simulink model "sysgenDDC"  (Simulink 7.7)
settings: Solver=VariableStepDiscrete  SolverMode=SingleTasking  StartTime=0.0  StopTime=0.003  RelTol=1e-3
PreLoadFcn:
  | sysgenDDC_PreLoadFcn
values from neighbouring files (symbols this model uses):
  Gz = [  340 ... (first row only)    [sysgenDDC_PreLoadFcn.m]
  Hz = [479 ... (first row only)    [sysgenDDC_PreLoadFcn.m]
  Ts = 1/40e006    (= 2.5e-08)    [sysgenDDC_PreLoadFcn.m]
undefined symbols (not defined in the file or in its folder): get, One, sided, xlGetSimulinkPeriod, xlipgetpartsetting
libraries: xbsIndex_r4 x132, dspsnks4 x2, xbsCopyrightNotice_r4 x1
(part 2 of 2)

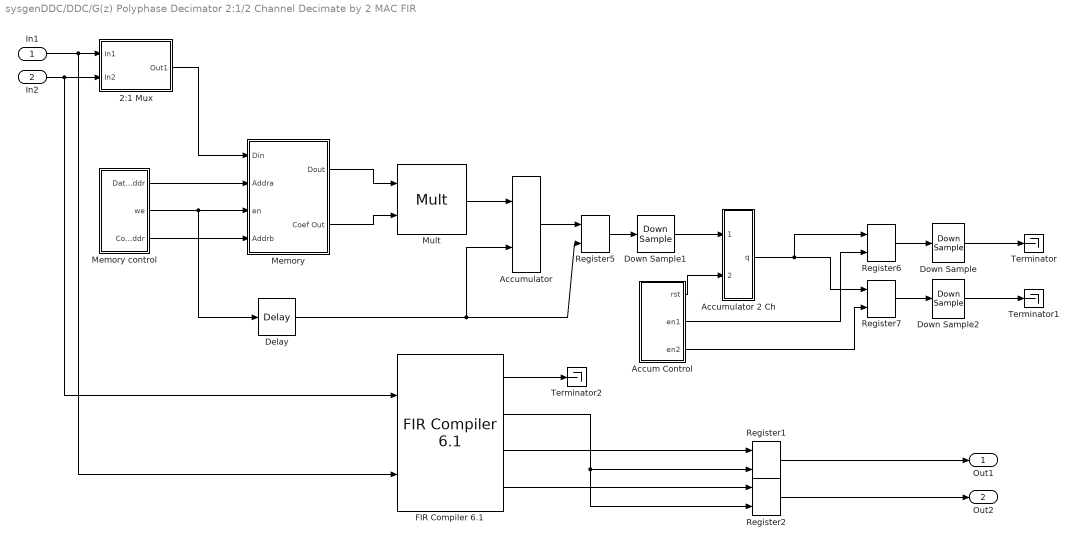
== system sysgenDDC/DDC/G(z) Polyphase Decimator 2:1/2 Channel Decimate by 2 MAC FIR  ==
  In1 : Inport
  In2 : Inport  Port=2
  2:1 Mux : Subsystem
  Accum Control : Subsystem
  Accumulator : xbsIndex_r4/Accumulator  operation=Add  n_bits=ceil(log2(coef_sum*(2^(bit_width-1))))  overflow=Wrap  scale=1  rst=on  hasbypass=on  en=off  dbl_ovrd=off  use_behavioral_HDL=on  implementation=Fabric  block_type=accum
      settings: infoedit="Adder or subtractor-based accumulator.   Output type and binary point position match the input.<P><P>Hardware notes: When \"Reinitialize with input 'b' on reset\" is selected, the accumulator is forced to run at the system rate even if the input 'b' is running at a slower rate."  xl_area=[18 36 0 36 0 0 0]  block_version=VER_STRING_GOES_HERE
  Accumulator 2 Ch : Subsystem
  Delay : xbsIndex_r4/Delay  rst=off  infoeditControl=Selection of Reset will increase slice count due to use of real FFs and instead of SRLs  en=off  latency=3  dbl_ovrd=off  reg_retiming=off  block_type=delay
      settings: infoedit=Hardware notes: A delay line is a chain, each link of which is an SRL16 followed by a flip-flop. If register retiming is enabled, the delay line is a chain of flip-flops.  xl_area=[1 1 0 1 0 0 0]  block_version=VER_STRING_GOES_HERE
  Down Sample : xbsIndex_r4/Down Sample  sample_ratio=4  sample_phase="Last Value of Frame  (most efficient)"  en=off  latency=1  dbl_ovrd=off  block_type=dsamp
      settings: xl_area=[19 37 0 0 0 0 0]  block_version=VER_STRING_GOES_HERE
  Down Sample1 : xbsIndex_r4/Down Sample  sample_ratio=length(coef)/4  sample_phase="Last Value of Frame  (most efficient)"  en=off  latency=1  dbl_ovrd=off  block_type=dsamp
      settings: xl_area=[18 36 0 0 0 0 0]  block_version=VER_STRING_GOES_HERE
  Down Sample2 : xbsIndex_r4/Down Sample  sample_ratio=4  sample_phase="Last Value of Frame  (most efficient)"  en=off  latency=1  dbl_ovrd=off  block_type=dsamp
      settings: xl_area=[19 37 0 0 0 0 0]  block_version=VER_STRING_GOES_HERE
  "FIR Compiler 6.1 " : xbsIndex_r4/FIR Compiler 6.1   coefficientvector=Gz  coefficient_sets=1  filter_type=Decimation  rate_change_type=Integer  interpolation_rate=1  decimation_rate=2  number_channels=1  ratespecification=Maximum_Possible  sampleperiod=96  hardwareoversamplingrate=1  coefficient_reload=off  coefficient_sign=Signed  quantization=Integer_Coefficients  coefficient_width=18  bestprecision=off  coefficient_fractional_bits=0  coefficient_structure=Inferred  number_paths=2  output_rounding_mode=Full_Precision  output_width=36  optimization_goal=Area  data_has_tlast=Not_Required  m_data_has_tready=off  s_data_has_tuser=Not_Required  m_data_has_tuser=Not_Required  s_config_sync_mode=On_Vector  s_config_method=Single  num_reload_slots=1  has_aclken=off  has_aresetn=off  multi_column_support=Disabled  columnconfig='7'  inter_column_pipe_length=4  data_buffer_type=Automatic  coefficient_buffer_type=Automatic  input_buffer_type=Automatic  output_buffer_type=Automatic  preference_for_other_storage=Automatic  trim_axipin_name=on  passband_min=0.0  passband_max=0.5  stopband_min=0.5  stopband_max=1.0  filter_selection=1  gui_behaviour=Sysgen_GUI  data_sign=Signed  data_width=16  data_fractional_bits=0  wrapper_available=true  ip_wrap_arbitrary_binary_point=true  ip_name=FIR Compiler  ip_version=6.1  dsptool_ready=true  ipcore_usecache=true  ipcore_useipmodelcache=true  ipcore_xco_need_fpga_part=true  port_translation_map={ 'aclken' => 'en', 'aresetn' => 'rst' }  run_core_at_system_period=true  ipcore_fpga_part=xlipgetpartsetting(gcb, {'virtex6', 'xc6vlx75t', '-3', 'ff784'})  structural_sim=false  block_type=fir_compiler_v6_1
      settings: infoedit=Maximum Possible : Maximizes oversampling rate. Abtracted input handshake (no s_data_tvalid) and automatic rate propagation.<br><br>Hardware Oversampling Rate : Specifies oversampling rate relative to the input sample period. Abtracted input handshake (no s_data_tvalid) and automatic rate propagation.<br><br>Sample Period : Specifies absolute oversampling rate. No input handshake abstraction (exposes s_data_tvalid) and no rate propagation.
  Memory : Subsystem
  Memory control : Subsystem
  Mult : xbsIndex_r4/Mult  precision=Full  arith_type="Signed  (2's comp)"  n_bits=8  bin_pt=2  quantization=Truncate  overflow=Wrap  en=off  latency=1  dbl_ovrd=off  use_behavioral_HDL=off  opt=Speed  use_embedded=on  optimum_pipeline=off  pipeline=on  use_rpm=off  placement_style=Rectangular shape  block_type=mult
      settings: infoedit=Hardware notes: To use the internal pipeline stage of the dedicated multiplier you must select 'Pipeline to Greatest Extent Possible'.  xl_area=[0 0 0 0 0 1 0]  block_version=VER_STRING_GOES_HERE
  Register{1..2,5..7} (5 alike) : xbsIndex_r4/Register  init=0  rst=off  en=on  dbl_ovrd=off  block_type=register
      Register1 settings: xl_area=[19 37 0 0 0 0 0]  block_version=VER_STRING_GOES_HERE
      Register2 settings: xl_area=[19 37 0 0 0 0 0]  block_version=VER_STRING_GOES_HERE
      Register5 settings: xl_area=[18 36 0 0 0 0 0]  block_version=VER_STRING_GOES_HERE
      Register6 settings: xl_area=[19 37 0 0 0 0 0]  block_version=VER_STRING_GOES_HERE
      Register7 settings: xl_area=[19 37 0 0 0 0 0]  block_version=VER_STRING_GOES_HERE
  Terminator : Terminator
  Terminator1 : Terminator
  Terminator2 : Terminator
  Out1 : Outport
  Out2 : Outport  Port=2
  wires:
  In2/1 -> 2:1 Mux/2(In2), "FIR Compiler 6.1 "/1
  Accum Control/3(en2) -> Register7/2
  Accum Control/2(en1) -> Register6/2
  Accum Control/1(rst) -> Accumulator 2 Ch/2(rst)
  Register7/1 -> Down Sample2/1
  Accumulator 2 Ch/1(q) -> Register6/1, Register7/1
  Register6/1 -> Down Sample/1
  Register5/1 -> Down Sample1/1
  Accumulator/1 -> Register5/1
  Memory control/3(Coef Addr) -> Memory/4(Addrb)
  Memory control/2(we) -> Delay/1, Memory/3(en)
  Memory control/1(Data Addr) -> Memory/2(Addra)
  Memory/1(Dout) -> Mult/1
  Mult/1 -> Accumulator/1
  Delay/1 -> Accumulator/2, Register5/2
  Down Sample1/1 -> Accumulator 2 Ch/1(In)
  Memory/2(Coef Out) -> Mult/2
  2:1 Mux/1(Out1) -> Memory/1(Din)
  In1/1 -> 2:1 Mux/1(In1), "FIR Compiler 6.1 "/2
  Register1/1 -> Out1/1
  Register2/1 -> Out2/1
  "FIR Compiler 6.1 "/4 -> Register2/1
  "FIR Compiler 6.1 "/3 -> Register1/1
  "FIR Compiler 6.1 "/2 -> Register1/2, Register2/2
  Down Sample/1 -> Terminator/1
  Down Sample2/1 -> Terminator1/1
  "FIR Compiler 6.1 "/1 -> Terminator2/1

== system sysgenDDC/DDC/G(z) Polyphase Decimator 2:1/Symmetric Round2 ==
  data : Inport
  Convert : xbsIndex_r4/Convert  gui_display_data_type=Fixed-point  arith_type="Signed  (2's comp)"  n_bits=18  bin_pt=0  float_type=Single  exp_bits=8  fraction_bits=24  quantization="Round  (unbiased: +/- Inf)"  overflow=Flag as error  en=off  latency=0  dbl_ovrd=off  pipeline=off  block_type=convert
      settings: xl_area=[13 0 0 25 0 0 0]  block_version=VER_STRING_GOES_HERE
  Reinterpret : xbsIndex_r4/Reinterpret  force_arith_type=off  arith_type="Signed  (2's comp)"  force_bin_pt=on  bin_pt=38-18  block_type=cast
      settings: infoedit="Changes signal type without altering the binary representation.   You can changed the signal between signed and unsigned, and relocate the binary point.<br><br>Hardware notes: In hardware this block costs nothing.<br><br>Example:  Suppose the input is 6 bits wide, signed, with 2 fractional bits, and the output is forced to unsigned with 0 fractional bits.  Then an input of -2.0 (1110.00 in binary 2's complement) becomes an output of 56 (111000 in binary)."  block_version=VER_STRING_GOES_HERE
  " out" : Outport
  wires:
  Reinterpret/1 -> Convert/1
  data/1 -> Reinterpret/1
  Convert/1 -> " out"/1

== system sysgenDDC/DDC/G(z) Polyphase Decimator 2:1/Symmetric Round3 ==
  data : Inport
  Convert : xbsIndex_r4/Convert  gui_display_data_type=Fixed-point  arith_type="Signed  (2's comp)"  n_bits=18  bin_pt=0  float_type=Single  exp_bits=8  fraction_bits=24  quantization="Round  (unbiased: +/- Inf)"  overflow=Flag as error  en=off  latency=0  dbl_ovrd=off  pipeline=off  block_type=convert
      settings: xl_area=[13 0 0 25 0 0 0]  block_version=VER_STRING_GOES_HERE
  Reinterpret : xbsIndex_r4/Reinterpret  force_arith_type=off  arith_type="Signed  (2's comp)"  force_bin_pt=on  bin_pt=38-18  block_type=cast
      settings: infoedit="Changes signal type without altering the binary representation.   You can changed the signal between signed and unsigned, and relocate the binary point.<br><br>Hardware notes: In hardware this block costs nothing.<br><br>Example:  Suppose the input is 6 bits wide, signed, with 2 fractional bits, and the output is forced to unsigned with 0 fractional bits.  Then an input of -2.0 (1110.00 in binary 2's complement) becomes an output of 56 (111000 in binary)."  block_version=VER_STRING_GOES_HERE
  " out" : Outport
  wires:
  Reinterpret/1 -> Convert/1
  Convert/1 -> " out"/1
  data/1 -> Reinterpret/1

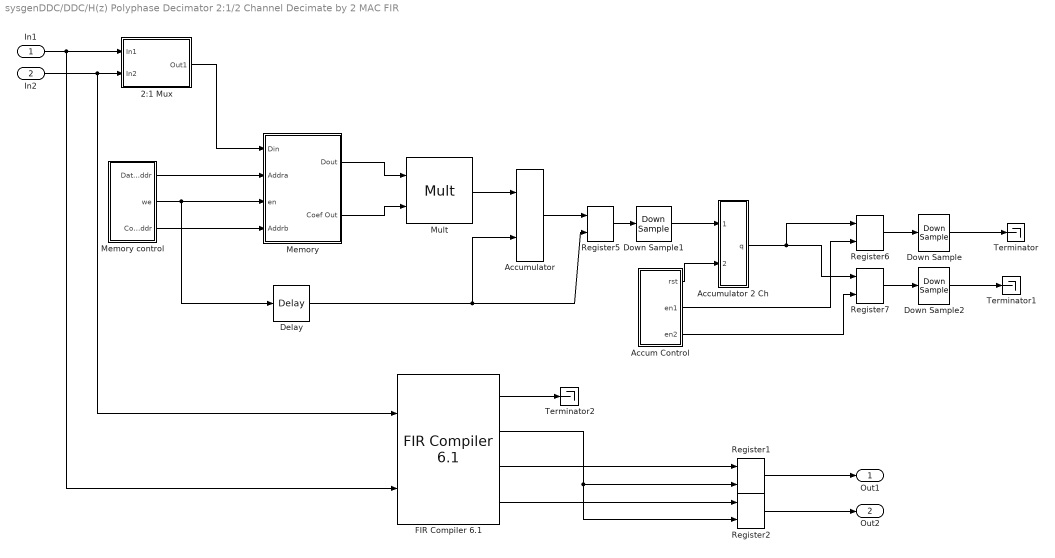
== system sysgenDDC/DDC/H(z) Polyphase Decimator 2:1/2 Channel Decimate by 2 MAC FIR  ==
  In1 : Inport
  In2 : Inport  Port=2
  2:1 Mux : Subsystem
  Accum Control : Subsystem
  Accumulator : xbsIndex_r4/Accumulator  operation=Add  n_bits=ceil(log2(coef_sum*(2^(bit_width-1))))  overflow=Wrap  scale=1  rst=on  hasbypass=on  en=off  dbl_ovrd=off  use_behavioral_HDL=on  implementation=Fabric  block_type=accum
      settings: infoedit="Adder or subtractor-based accumulator.   Output type and binary point position match the input.<P><P>Hardware notes: When \"Reinitialize with input 'b' on reset\" is selected, the accumulator is forced to run at the system rate even if the input 'b' is running at a slower rate."  xl_area=[18 36 0 36 0 0 0]  block_version=VER_STRING_GOES_HERE
  Accumulator 2 Ch : Subsystem
  Delay : xbsIndex_r4/Delay  rst=off  infoeditControl=Selection of Reset will increase slice count due to use of real FFs and instead of SRLs  en=off  latency=4  dbl_ovrd=off  reg_retiming=off  block_type=delay
      settings: infoedit=Hardware notes: A delay line is a chain, each link of which is an SRL16 followed by a flip-flop. If register retiming is enabled, the delay line is a chain of flip-flops.  xl_area=[1 1 0 1 0 0 0]  block_version=VER_STRING_GOES_HERE
  Down Sample : xbsIndex_r4/Down Sample  sample_ratio=4  sample_phase="Last Value of Frame  (most efficient)"  en=off  latency=1  dbl_ovrd=off  block_type=dsamp
      settings: xl_area=[19 37 0 0 0 0 0]  block_version=VER_STRING_GOES_HERE
  Down Sample1 : xbsIndex_r4/Down Sample  sample_ratio=length(coef)/4  sample_phase="Last Value of Frame  (most efficient)"  en=off  latency=1  dbl_ovrd=off  block_type=dsamp
      settings: xl_area=[18 36 0 0 0 0 0]  block_version=VER_STRING_GOES_HERE
  Down Sample2 : xbsIndex_r4/Down Sample  sample_ratio=4  sample_phase="Last Value of Frame  (most efficient)"  en=off  latency=1  dbl_ovrd=off  block_type=dsamp
      settings: xl_area=[19 37 0 0 0 0 0]  block_version=VER_STRING_GOES_HERE
  "FIR Compiler 6.1 " : xbsIndex_r4/FIR Compiler 6.1   coefficientvector=Hz  coefficient_sets=1  filter_type=Decimation  rate_change_type=Integer  interpolation_rate=1  decimation_rate=2  number_channels=1  ratespecification=Maximum_Possible  sampleperiod=96  hardwareoversamplingrate=1  coefficient_reload=off  coefficient_sign=Signed  quantization=Integer_Coefficients  coefficient_width=18  bestprecision=off  coefficient_fractional_bits=0  coefficient_structure=Inferred  number_paths=2  output_rounding_mode=Full_Precision  output_width=36  optimization_goal=Area  data_has_tlast=Not_Required  m_data_has_tready=off  s_data_has_tuser=Not_Required  m_data_has_tuser=Not_Required  s_config_sync_mode=On_Vector  s_config_method=Single  num_reload_slots=1  has_aclken=off  has_aresetn=off  multi_column_support=Disabled  columnconfig='26'  inter_column_pipe_length=4  data_buffer_type=Automatic  coefficient_buffer_type=Automatic  input_buffer_type=Automatic  output_buffer_type=Automatic  preference_for_other_storage=Automatic  trim_axipin_name=on  passband_min=0.0  passband_max=0.5  stopband_min=0.5  stopband_max=1.0  filter_selection=1  gui_behaviour=Sysgen_GUI  data_sign=Signed  data_width=16  data_fractional_bits=0  wrapper_available=true  ip_wrap_arbitrary_binary_point=true  ip_name=FIR Compiler  ip_version=6.1  dsptool_ready=true  ipcore_usecache=true  ipcore_useipmodelcache=true  ipcore_xco_need_fpga_part=true  port_translation_map={ 'aclken' => 'en', 'aresetn' => 'rst' }  run_core_at_system_period=true  ipcore_fpga_part=xlipgetpartsetting(gcb, {'virtex6', 'xc6vlx75t', '-3', 'ff784'})  structural_sim=false  block_type=fir_compiler_v6_1
      settings: infoedit=Maximum Possible : Maximizes oversampling rate. Abtracted input handshake (no s_data_tvalid) and automatic rate propagation.<br><br>Hardware Oversampling Rate : Specifies oversampling rate relative to the input sample period. Abtracted input handshake (no s_data_tvalid) and automatic rate propagation.<br><br>Sample Period : Specifies absolute oversampling rate. No input handshake abstraction (exposes s_data_tvalid) and no rate propagation.
  Memory : Subsystem
  Memory control : Subsystem
  Mult : xbsIndex_r4/Mult  precision=Full  arith_type="Signed  (2's comp)"  n_bits=8  bin_pt=2  quantization=Truncate  overflow=Wrap  en=off  latency=2  dbl_ovrd=off  use_behavioral_HDL=off  opt=Speed  use_embedded=on  optimum_pipeline=off  pipeline=on  use_rpm=off  placement_style=Rectangular shape  block_type=mult
      settings: infoedit=Hardware notes: To use the internal pipeline stage of the dedicated multiplier you must select 'Pipeline to Greatest Extent Possible'.  xl_area=[18 36 0 0 0 1 0]  block_version=VER_STRING_GOES_HERE
  Register{1..2,5..7} (5 alike) : xbsIndex_r4/Register  init=0  rst=off  en=on  dbl_ovrd=off  block_type=register
      Register1 settings: xl_area=[19 37 0 0 0 0 0]  block_version=VER_STRING_GOES_HERE
      Register2 settings: xl_area=[19 37 0 0 0 0 0]  block_version=VER_STRING_GOES_HERE
      Register5 settings: xl_area=[18 36 0 0 0 0 0]  block_version=VER_STRING_GOES_HERE
      Register6 settings: xl_area=[19 37 0 0 0 0 0]  block_version=VER_STRING_GOES_HERE
      Register7 settings: xl_area=[19 37 0 0 0 0 0]  block_version=VER_STRING_GOES_HERE
  Terminator : Terminator
  Terminator1 : Terminator
  Terminator2 : Terminator
  Out1 : Outport
  Out2 : Outport  Port=2
  wires:
  In1/1 -> 2:1 Mux/1(In1), "FIR Compiler 6.1 "/2
  2:1 Mux/1(Out1) -> Memory/1(Din)
  Memory/2(Coef Out) -> Mult/2
  Down Sample1/1 -> Accumulator 2 Ch/1(In)
  Delay/1 -> Register5/2, Accumulator/2
  Mult/1 -> Accumulator/1
  Memory/1(Dout) -> Mult/1
  Memory control/1(Data Addr) -> Memory/2(Addra)
  Memory control/2(we) -> Memory/3(en), Delay/1
  Memory control/3(Coef Addr) -> Memory/4(Addrb)
  Accumulator/1 -> Register5/1
  Register5/1 -> Down Sample1/1
  Register6/1 -> Down Sample/1
  Accumulator 2 Ch/1(q) -> Register7/1, Register6/1
  Register7/1 -> Down Sample2/1
  Accum Control/1(rst) -> Accumulator 2 Ch/2(rst)
  Accum Control/2(en1) -> Register6/2
  Accum Control/3(en2) -> Register7/2
  In2/1 -> 2:1 Mux/2(In2), "FIR Compiler 6.1 "/1
  "FIR Compiler 6.1 "/4 -> Register2/1
  "FIR Compiler 6.1 "/3 -> Register1/1
  "FIR Compiler 6.1 "/2 -> Register1/2, Register2/2
  Register1/1 -> Out1/1
  Register2/1 -> Out2/1
  Down Sample/1 -> Terminator/1
  Down Sample2/1 -> Terminator1/1
  "FIR Compiler 6.1 "/1 -> Terminator2/1

== system sysgenDDC/DDC/H(z) Polyphase Decimator 2:1/Coarse Gain ==
  data : Inport
  Reinterpret : xbsIndex_r4/Reinterpret  force_arith_type=on  arith_type="Signed  (2's comp)"  force_bin_pt=on  bin_pt=24  block_type=cast
      settings: infoedit="Changes type of samples without altering their binary representation.<P><P>Hardware notes: In hardware this block costs nothing.<P><P>Example:  Suppose the input is 6 bits wide, signed, with 2 fractional bits, and the output is forced to unsigned with 0 fractional bits.  Then an input of -2.0 (1110.00 in binary 2's complement) becomes an output of 56 (111000 in binary)."  block_version=VER_STRING_GOES_HERE
  Slice : xbsIndex_r4/Slice  nbits=26  boolean_output=off  mode=Upper Bit Location + Width  bit1=0  base1=MSB of Input  bit0=0  base0=LSB of Input  dbl_ovrd=off  block_type=slice
      settings: infoedit="Extracts a given range of bits from each input sample and presents it at the output.  The output type is ordinarily unsigned with binary point at zero, but can be Boolean when the slice is one bit wide.<P><P>Hardware notes: In hardware this block costs nothing."  block_version=VER_STRING_GOES_HERE
  " out" : Outport
  wires:
  Reinterpret/1 -> " out"/1
  Slice/1 -> Reinterpret/1
  data/1 -> Slice/1

== system sysgenDDC/DDC/H(z) Polyphase Decimator 2:1/Coarse Gain1 ==
  data : Inport
  Reinterpret : xbsIndex_r4/Reinterpret  force_arith_type=on  arith_type="Signed  (2's comp)"  force_bin_pt=on  bin_pt=24  block_type=cast
      settings: infoedit="Changes type of samples without altering their binary representation.<P><P>Hardware notes: In hardware this block costs nothing.<P><P>Example:  Suppose the input is 6 bits wide, signed, with 2 fractional bits, and the output is forced to unsigned with 0 fractional bits.  Then an input of -2.0 (1110.00 in binary 2's complement) becomes an output of 56 (111000 in binary)."  block_version=VER_STRING_GOES_HERE
  Slice : xbsIndex_r4/Slice  nbits=26  boolean_output=off  mode=Upper Bit Location + Width  bit1=0  base1=MSB of Input  bit0=0  base0=LSB of Input  dbl_ovrd=off  block_type=slice
      settings: infoedit="Extracts a given range of bits from each input sample and presents it at the output.  The output type is ordinarily unsigned with binary point at zero, but can be Boolean when the slice is one bit wide.<P><P>Hardware notes: In hardware this block costs nothing."  block_version=VER_STRING_GOES_HERE
  " out" : Outport
  wires:
  data/1 -> Slice/1
  Slice/1 -> Reinterpret/1
  Reinterpret/1 -> " out"/1

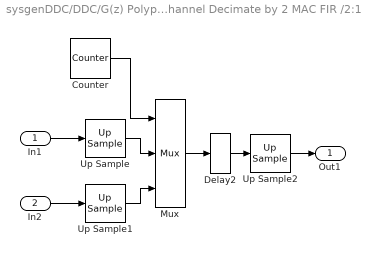
== system sysgenDDC/DDC/G(z) Polyphase Decimator 2:1/2 Channel Decimate by 2 MAC FIR /2:1 Mux ==
  In1 : Inport
  In2 : Inport  Port=2
  Counter : xbsIndex_r4/Counter  cnt_type=Free Running  cnt_to=Inf  operation=Up  start_count=0  cnt_by_val=1  arith_type=Unsigned  n_bits=1  bin_pt=0  load_pin=off  rst=off  en=off  explicit_period=off  period=Ts/2  dbl_ovrd=off  use_behavioral_HDL=off  implementation=Fabric  use_rpm=off  block_type=counter
      settings: xl_area=[2 1 0 1 0 0 0]  block_version=VER_STRING_GOES_HERE
  Delay2 : xbsIndex_r4/Delay  rst=off  infoeditControl=Selection of Reset will increase slice count due to use of real FFs and instead of SRLs  en=off  latency=1  dbl_ovrd=off  reg_retiming=off  block_type=delay
      settings: infoedit=Hardware notes: A delay line is a chain, each link of which is an SRL16 followed by a flip-flop. If register retiming is enabled, the delay line is a chain of flip-flops.  xl_area=[9 18 0 0 0 0 0]  block_version=VER_STRING_GOES_HERE
  Mux : xbsIndex_r4/Mux  inputs=2  en=off  latency=0  precision=Full  arith_type="Signed  (2's comp)"  n_bits=8  bin_pt=2  quantization=Truncate  overflow=Wrap  dbl_ovrd=off  block_type=mux
      settings: xl_area=[9 0 0 18 0 0 0]  block_version=VER_STRING_GOES_HERE
  Up Sample : xbsIndex_r4/Up Sample  sample_ratio=2  copy_samples=on  en=off  latency=0  dbl_ovrd=off  block_type=usamp
      settings: infoedit="Up samples input data.  Inserted values  can be zeros or copies of the most recent input sample.<P><P>Hardware notes: No hardware is needed if inserted values are copies of the input sample; otherwise, a mux and single bit flip-flop are used."  xl_area=[0 0 0 0 0 0 0]  block_version=VER_STRING_GOES_HERE
  Up Sample1 : xbsIndex_r4/Up Sample  sample_ratio=2  copy_samples=on  en=off  latency=0  dbl_ovrd=off  block_type=usamp
      settings: infoedit="Up samples input data.  Inserted values  can be zeros or copies of the most recent input sample.<P><P>Hardware notes: No hardware is needed if inserted values are copies of the input sample; otherwise, a mux and single bit flip-flop are used."  xl_area=[0 0 0 0 0 0 0]  block_version=VER_STRING_GOES_HERE
  Up Sample2 : xbsIndex_r4/Up Sample  sample_ratio=length(coef)/4  copy_samples=on  en=off  latency=0  dbl_ovrd=off  block_type=usamp
      settings: infoedit="Up samples input data.  Inserted values  can be zeros or copies of the most recent input sample.<P><P>Hardware notes: No hardware is needed if inserted values are copies of the input sample; otherwise, a mux and single bit flip-flop are used."  xl_area=[0 0 0 0 0 0 0]  block_version=VER_STRING_GOES_HERE
  Out1 : Outport
  wires:
  Up Sample2/1 -> Out1/1
  In2/1 -> Up Sample1/1
  In1/1 -> Up Sample/1
  Delay2/1 -> Up Sample2/1
  Mux/1 -> Delay2/1
  Counter/1 -> Mux/1
  Up Sample1/1 -> Mux/3
  Up Sample/1 -> Mux/2

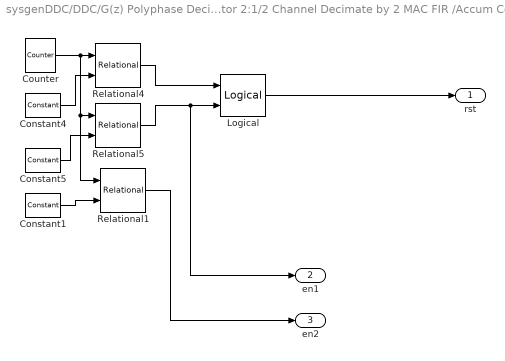
== system sysgenDDC/DDC/G(z) Polyphase Decimator 2:1/2 Channel Decimate by 2 MAC FIR /Accum Control ==
  Constant1 : xbsIndex_r4/Constant  const=2  gui_display_data_type=Fixed-point  arith_type=Unsigned  n_bits=2  bin_pt=0  preci_type=Single  exp_width=8  frac_width=24  explicit_period=off  period=1  equ=P=C  opselect=C  inp2=PCIN>>17  opr=+  inp1=P  carry=CIN  dbl_ovrd=off  block_type=constant
      settings: block_version=VER_STRING_GOES_HERE
  Constant4 : xbsIndex_r4/Constant  const=0  gui_display_data_type=Fixed-point  arith_type=Unsigned  n_bits=2  bin_pt=0  preci_type=Single  exp_width=8  frac_width=24  explicit_period=off  period=1  equ=P=C  opselect=C  inp2=PCIN>>17  opr=+  inp1=P  carry=CIN  dbl_ovrd=off  block_type=constant
      settings: block_version=VER_STRING_GOES_HERE
  Constant5 : xbsIndex_r4/Constant  const=1  gui_display_data_type=Fixed-point  arith_type=Unsigned  n_bits=2  bin_pt=0  preci_type=Single  exp_width=8  frac_width=24  explicit_period=off  period=1  equ=P=C  opselect=C  inp2=PCIN>>17  opr=+  inp1=P  carry=CIN  dbl_ovrd=off  block_type=constant
      settings: block_version=VER_STRING_GOES_HERE
  Counter : xbsIndex_r4/Counter  cnt_type=Free Running  cnt_to=Inf  operation=Up  start_count=0  cnt_by_val=1  arith_type=Unsigned  n_bits=2  bin_pt=0  load_pin=off  rst=off  en=off  explicit_period=off  period=Ts/2  dbl_ovrd=off  use_behavioral_HDL=off  implementation=Fabric  use_rpm=off  block_type=counter
      settings: xl_area=[1 2 0 2 0 0 0]  block_version=VER_STRING_GOES_HERE
  Logical : xbsIndex_r4/Logical  logical_function=OR  inputs=2  en=off  latency=0  precision=Full  arith_type=Unsigned  n_bits=8  bin_pt=2  align_bp=on  dbl_ovrd=off  block_type=logical
      settings: xl_area=[1 0 0 1 0 0 0]  block_version=VER_STRING_GOES_HERE
  Relational1 : xbsIndex_r4/Relational  mode=a=b  en=off  latency=0  dbl_ovrd=off  block_type=relational
      settings: xl_area=[1 0 0 1 0 0 0]  block_version=VER_STRING_GOES_HERE
  Relational4 : xbsIndex_r4/Relational  mode=a=b  en=off  latency=0  dbl_ovrd=off  block_type=relational
      settings: xl_area=[1 0 0 1 0 0 0]  block_version=VER_STRING_GOES_HERE
  Relational5 : xbsIndex_r4/Relational  mode=a=b  en=off  latency=0  dbl_ovrd=off  block_type=relational
      settings: xl_area=[1 0 0 1 0 0 0]  block_version=VER_STRING_GOES_HERE
  rst : Outport
  en1 : Outport  Port=2
  en2 : Outport  Port=3
  wires:
  Relational1/1 -> en2/1
  Constant1/1 -> Relational1/2
  Logical/1 -> rst/1
  Relational5/1 -> en1/1, Logical/2
  Relational4/1 -> Logical/1
  Constant5/1 -> Relational5/2
  Constant4/1 -> Relational4/2
  Counter/1 -> Relational1/1, Relational5/1, Relational4/1

== system sysgenDDC/DDC/G(z) Polyphase Decimator 2:1/2 Channel Decimate by 2 MAC FIR /Accumulator 2 Ch ==
  note: Active Low Reset
  In : Inport
  rst : Inport  Port=2
  AddSub : xbsIndex_r4/AddSub  mode=Addition  use_carryin=off  use_carryout=off  en=off  latency=0  precision=User Defined  arith_type="Signed  (2's comp)"  n_bits=ceil(log2(coef_sum*(2^(bit_width-1))))+1  bin_pt=0  quantization=Truncate  overflow=Wrap  dbl_ovrd=off  use_behavioral_HDL=on  hw_selection=Fabric  pipelined=off  use_rpm=off  block_type=addsub
      settings: xl_area=[19 0 0 37 0 0 0]  block_version=VER_STRING_GOES_HERE
  Delay : xbsIndex_r4/Delay  rst=off  infoeditControl=Selection of Reset will increase slice count due to use of real FFs and instead of SRLs  en=off  latency=1  dbl_ovrd=off  reg_retiming=off  block_type=delay
      settings: infoedit=Hardware notes: A delay line is a chain, each link of which is an SRL16 followed by a flip-flop. If register retiming is enabled, the delay line is a chain of flip-flops.  xl_area=[19 37 0 0 0 0 0]  block_version=VER_STRING_GOES_HERE
  Mux : xbsIndex_r4/Mux  inputs=2  en=off  latency=0  precision=Full  arith_type="Signed  (2's comp)"  n_bits=8  bin_pt=2  quantization=Truncate  overflow=Wrap  dbl_ovrd=off  block_type=mux
      settings: xl_area=[19 0 0 37 0 0 0]  block_version=VER_STRING_GOES_HERE
  Register : xbsIndex_r4/Register  init=0  rst=off  en=off  dbl_ovrd=off  block_type=register
      settings: xl_area=[19 37 0 0 0 0 0]  block_version=VER_STRING_GOES_HERE
  q : Outport
  wires:
  Delay/1 -> AddSub/2
  Register/1 -> q/1, Delay/1
  Mux/1 -> Register/1
  AddSub/1 -> Mux/3
  rst/1 -> Mux/1
  In/1 -> Mux/2, AddSub/1

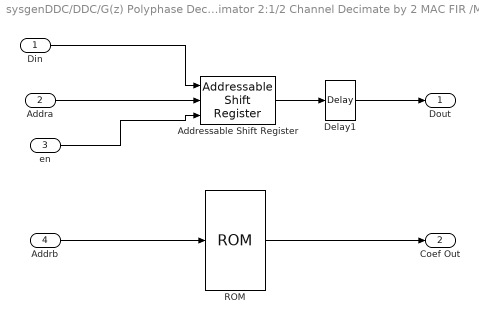
== system sysgenDDC/DDC/G(z) Polyphase Decimator 2:1/2 Channel Decimate by 2 MAC FIR /Memory ==
  Din : Inport
  Addra : Inport  Port=2
  en : Inport  Port=3
  Addrb : Inport  Port=4
  Addressable Shift Register : xbsIndex_r4/Addressable Shift Register  infer_latency=on  depth=2  initVector=[0]  en=on  dbl_ovrd=off  use_behavioral_HDL=off  Optimization=Resource  use_rpm=off  block_type=addrsr
      settings: infoedit="Delay of  configurable length.  Any element  in the delay     line   can    be   addressed   and   driven    onto   the   output     port.<P><P>Hardware  notes: Implemented  using SRL16s.     If Virtex-4, Virtex-II or Spartan-3 devices are used, multiple SRLC16s are cascaded together."  xl_area=[54 0 0 108 0 0 0]  block_version=VER_STRING_GOES_HERE
  Delay1 : xbsIndex_r4/Delay  rst=off  infoeditControl=Selection of Reset will increase slice count due to use of real FFs and instead of SRLs  en=off  latency=1  dbl_ovrd=off  reg_retiming=off  block_type=delay
      settings: infoedit=Hardware notes: A delay line is a chain, each link of which is an SRL16 followed by a flip-flop. If register retiming is enabled, the delay line is a chain of flip-flops.  xl_area=[9 18 0 0 0 0 0]  block_version=VER_STRING_GOES_HERE
  ROM : xbsIndex_r4/ROM  depth=length(coef)  initVector=coef  distributed_mem=Block RAM  rst=off  init_reg=0  en=off  latency=1  gui_display_data_type=Fixed-point  arith_type="Signed  (2's comp)"  n_bits=coef_bit_width  bin_pt=coef_bin_pt  preci_type=Single  exp_width=8  frac_width=24  dbl_ovrd=off  optimize=Area  use_rpm=off  block_type=sprom
      settings: xl_area=[0 0 1 0 0 0 0]  block_version=VER_STRING_GOES_HERE
  Dout : Outport
  Coef Out : Outport  Port=2
  wires:
  Delay1/1 -> Dout/1
  ROM/1 -> Coef Out/1
  Addrb/1 -> ROM/1
  Addressable Shift Register/1 -> Delay1/1
  Addra/1 -> Addressable Shift Register/2
  Din/1 -> Addressable Shift Register/1
  en/1 -> Addressable Shift Register/3

== system sysgenDDC/DDC/G(z) Polyphase Decimator 2:1/2 Channel Decimate by 2 MAC FIR /Memory control ==
  Constant : xbsIndex_r4/Constant  const=length(coef)-4  gui_display_data_type=Fixed-point  arith_type=Unsigned  n_bits=ceil(log2(length(coef)-4))  bin_pt=0  preci_type=Single  exp_width=8  frac_width=24  explicit_period=off  period=1  equ=P=C  opselect=C  inp2=PCIN>>17  opr=+  inp1=P  carry=CIN  dbl_ovrd=off  block_type=constant
      settings: block_version=VER_STRING_GOES_HERE
  Counter1 : xbsIndex_r4/Counter  cnt_type=Count Limited  cnt_to=length(coef)-4  operation=Up  start_count=0  cnt_by_val=4  arith_type=Unsigned  n_bits=ceil(log2(length(coef)-1))  bin_pt=0  load_pin=off  rst=off  en=off  explicit_period=on  period=Ts/(length(coef)/2)  dbl_ovrd=off  use_behavioral_HDL=off  implementation=Fabric  use_rpm=off  block_type=counter
      settings: xl_area=[4 6 0 8 0 0 0]  block_version=VER_STRING_GOES_HERE
  Counter2 : xbsIndex_r4/Counter  cnt_type=Count Limited  cnt_to=length(coef)-1  operation=Up  start_count=0  cnt_by_val=1  arith_type=Unsigned  n_bits=ceil(log2(length(coef)-1))  bin_pt=0  load_pin=off  rst=off  en=off  explicit_period=off  period=Ts/(length(coef)/2)  dbl_ovrd=off  use_behavioral_HDL=off  implementation=Fabric  use_rpm=off  block_type=counter
      settings: xl_area=[4 6 0 8 0 0 0]  block_version=VER_STRING_GOES_HERE
  Relational : xbsIndex_r4/Relational  mode=a=b  en=off  latency=0  dbl_ovrd=off  block_type=relational
      settings: xl_area=[2 0 0 3 0 0 0]  block_version=VER_STRING_GOES_HERE
  Data Addr : Outport
  we : Outport  Port=2
  Coef Addr : Outport  Port=3
  wires:
  Counter2/1 -> Coef Addr/1
  Relational/1 -> we/1
  Constant/1 -> Relational/2
  Counter1/1 -> Data Addr/1, Relational/1

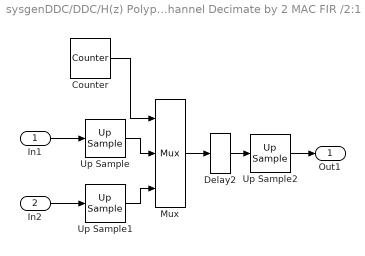
== system sysgenDDC/DDC/H(z) Polyphase Decimator 2:1/2 Channel Decimate by 2 MAC FIR /2:1 Mux ==
  In1 : Inport
  In2 : Inport  Port=2
  Counter : xbsIndex_r4/Counter  cnt_type=Free Running  cnt_to=Inf  operation=Up  start_count=0  cnt_by_val=1  arith_type=Unsigned  n_bits=1  bin_pt=0  load_pin=off  rst=off  en=off  explicit_period=off  period=Ts/2  dbl_ovrd=off  use_behavioral_HDL=off  implementation=Fabric  use_rpm=off  block_type=counter
      settings: xl_area=[2 1 0 1 0 0 0]  block_version=VER_STRING_GOES_HERE
  Delay2 : xbsIndex_r4/Delay  rst=off  infoeditControl=Selection of Reset will increase slice count due to use of real FFs and instead of SRLs  en=off  latency=1  dbl_ovrd=off  reg_retiming=off  block_type=delay
      settings: infoedit=Hardware notes: A delay line is a chain, each link of which is an SRL16 followed by a flip-flop. If register retiming is enabled, the delay line is a chain of flip-flops.  xl_area=[9 18 0 0 0 0 0]  block_version=VER_STRING_GOES_HERE
  Mux : xbsIndex_r4/Mux  inputs=2  en=off  latency=0  precision=Full  arith_type="Signed  (2's comp)"  n_bits=8  bin_pt=2  quantization=Truncate  overflow=Wrap  dbl_ovrd=off  block_type=mux
      settings: xl_area=[9 0 0 18 0 0 0]  block_version=VER_STRING_GOES_HERE
  Up Sample : xbsIndex_r4/Up Sample  sample_ratio=2  copy_samples=on  en=off  latency=0  dbl_ovrd=off  block_type=usamp
      settings: infoedit="Up samples input data.  Inserted values  can be zeros or copies of the most recent input sample.<P><P>Hardware notes: No hardware is needed if inserted values are copies of the input sample; otherwise, a mux and single bit flip-flop are used."  xl_area=[0 0 0 0 0 0 0]  block_version=VER_STRING_GOES_HERE
  Up Sample1 : xbsIndex_r4/Up Sample  sample_ratio=2  copy_samples=on  en=off  latency=0  dbl_ovrd=off  block_type=usamp
      settings: infoedit="Up samples input data.  Inserted values  can be zeros or copies of the most recent input sample.<P><P>Hardware notes: No hardware is needed if inserted values are copies of the input sample; otherwise, a mux and single bit flip-flop are used."  xl_area=[0 0 0 0 0 0 0]  block_version=VER_STRING_GOES_HERE
  Up Sample2 : xbsIndex_r4/Up Sample  sample_ratio=length(coef)/4  copy_samples=on  en=off  latency=0  dbl_ovrd=off  block_type=usamp
      settings: infoedit="Up samples input data.  Inserted values  can be zeros or copies of the most recent input sample.<P><P>Hardware notes: No hardware is needed if inserted values are copies of the input sample; otherwise, a mux and single bit flip-flop are used."  xl_area=[0 0 0 0 0 0 0]  block_version=VER_STRING_GOES_HERE
  Out1 : Outport
  wires:
  Up Sample/1 -> Mux/2
  Up Sample1/1 -> Mux/3
  Counter/1 -> Mux/1
  Mux/1 -> Delay2/1
  Delay2/1 -> Up Sample2/1
  In1/1 -> Up Sample/1
  In2/1 -> Up Sample1/1
  Up Sample2/1 -> Out1/1

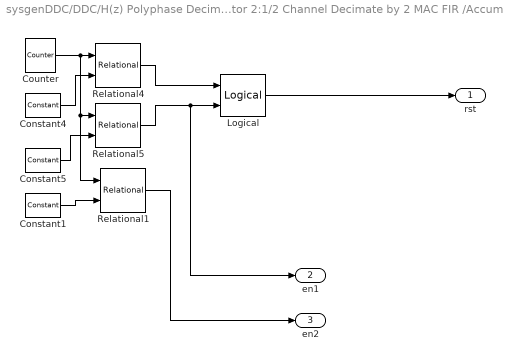
== system sysgenDDC/DDC/H(z) Polyphase Decimator 2:1/2 Channel Decimate by 2 MAC FIR /Accum Control ==
  Constant1 : xbsIndex_r4/Constant  const=2  gui_display_data_type=Fixed-point  arith_type=Unsigned  n_bits=2  bin_pt=0  preci_type=Single  exp_width=8  frac_width=24  explicit_period=off  period=1  equ=P=C  opselect=C  inp2=PCIN>>17  opr=+  inp1=P  carry=CIN  dbl_ovrd=off  block_type=constant
      settings: block_version=VER_STRING_GOES_HERE
  Constant4 : xbsIndex_r4/Constant  const=0  gui_display_data_type=Fixed-point  arith_type=Unsigned  n_bits=2  bin_pt=0  preci_type=Single  exp_width=8  frac_width=24  explicit_period=off  period=1  equ=P=C  opselect=C  inp2=PCIN>>17  opr=+  inp1=P  carry=CIN  dbl_ovrd=off  block_type=constant
      settings: block_version=VER_STRING_GOES_HERE
  Constant5 : xbsIndex_r4/Constant  const=1  gui_display_data_type=Fixed-point  arith_type=Unsigned  n_bits=2  bin_pt=0  preci_type=Single  exp_width=8  frac_width=24  explicit_period=off  period=1  equ=P=C  opselect=C  inp2=PCIN>>17  opr=+  inp1=P  carry=CIN  dbl_ovrd=off  block_type=constant
      settings: block_version=VER_STRING_GOES_HERE
  Counter : xbsIndex_r4/Counter  cnt_type=Free Running  cnt_to=Inf  operation=Up  start_count=0  cnt_by_val=1  arith_type=Unsigned  n_bits=2  bin_pt=0  load_pin=off  rst=off  en=off  explicit_period=off  period=Ts/2  dbl_ovrd=off  use_behavioral_HDL=off  implementation=Fabric  use_rpm=off  block_type=counter
      settings: xl_area=[1 2 0 2 0 0 0]  block_version=VER_STRING_GOES_HERE
  Logical : xbsIndex_r4/Logical  logical_function=OR  inputs=2  en=off  latency=0  precision=Full  arith_type=Unsigned  n_bits=8  bin_pt=2  align_bp=on  dbl_ovrd=off  block_type=logical
      settings: xl_area=[1 0 0 1 0 0 0]  block_version=VER_STRING_GOES_HERE
  Relational1 : xbsIndex_r4/Relational  mode=a=b  en=off  latency=0  dbl_ovrd=off  block_type=relational
      settings: xl_area=[1 0 0 1 0 0 0]  block_version=VER_STRING_GOES_HERE
  Relational4 : xbsIndex_r4/Relational  mode=a=b  en=off  latency=0  dbl_ovrd=off  block_type=relational
      settings: xl_area=[1 0 0 1 0 0 0]  block_version=VER_STRING_GOES_HERE
  Relational5 : xbsIndex_r4/Relational  mode=a=b  en=off  latency=0  dbl_ovrd=off  block_type=relational
      settings: xl_area=[1 0 0 1 0 0 0]  block_version=VER_STRING_GOES_HERE
  rst : Outport
  en1 : Outport  Port=2
  en2 : Outport  Port=3
  wires:
  Counter/1 -> Relational4/1, Relational5/1, Relational1/1
  Constant4/1 -> Relational4/2
  Constant5/1 -> Relational5/2
  Relational4/1 -> Logical/1
  Relational5/1 -> Logical/2, en1/1
  Logical/1 -> rst/1
  Constant1/1 -> Relational1/2
  Relational1/1 -> en2/1

== system sysgenDDC/DDC/H(z) Polyphase Decimator 2:1/2 Channel Decimate by 2 MAC FIR /Accumulator 2 Ch ==
  note: Active Low Reset
  In : Inport
  rst : Inport  Port=2
  AddSub : xbsIndex_r4/AddSub  mode=Addition  use_carryin=off  use_carryout=off  en=off  latency=0  precision=User Defined  arith_type="Signed  (2's comp)"  n_bits=ceil(log2(coef_sum*(2^(bit_width-1))))+1  bin_pt=0  quantization=Truncate  overflow=Wrap  dbl_ovrd=off  use_behavioral_HDL=on  hw_selection=Fabric  pipelined=off  use_rpm=off  block_type=addsub
      settings: xl_area=[19 0 0 37 0 0 0]  block_version=VER_STRING_GOES_HERE
  Delay : xbsIndex_r4/Delay  rst=off  infoeditControl=Selection of Reset will increase slice count due to use of real FFs and instead of SRLs  en=off  latency=1  dbl_ovrd=off  reg_retiming=off  block_type=delay
      settings: infoedit=Hardware notes: A delay line is a chain, each link of which is an SRL16 followed by a flip-flop. If register retiming is enabled, the delay line is a chain of flip-flops.  xl_area=[19 37 0 0 0 0 0]  block_version=VER_STRING_GOES_HERE
  Mux : xbsIndex_r4/Mux  inputs=2  en=off  latency=0  precision=Full  arith_type="Signed  (2's comp)"  n_bits=8  bin_pt=2  quantization=Truncate  overflow=Wrap  dbl_ovrd=off  block_type=mux
      settings: xl_area=[19 0 0 37 0 0 0]  block_version=VER_STRING_GOES_HERE
  Register : xbsIndex_r4/Register  init=0  rst=off  en=off  dbl_ovrd=off  block_type=register
      settings: xl_area=[19 37 0 0 0 0 0]  block_version=VER_STRING_GOES_HERE
  q : Outport
  wires:
  In/1 -> AddSub/1, Mux/2
  rst/1 -> Mux/1
  AddSub/1 -> Mux/3
  Mux/1 -> Register/1
  Register/1 -> Delay/1, q/1
  Delay/1 -> AddSub/2

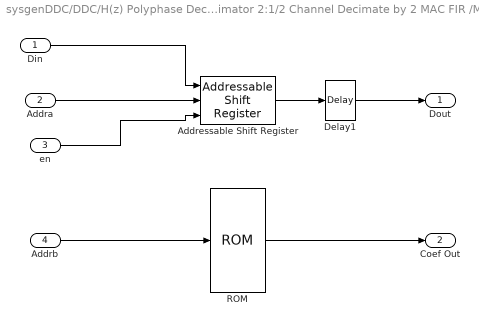
== system sysgenDDC/DDC/H(z) Polyphase Decimator 2:1/2 Channel Decimate by 2 MAC FIR /Memory ==
  Din : Inport
  Addra : Inport  Port=2
  en : Inport  Port=3
  Addrb : Inport  Port=4
  Addressable Shift Register : xbsIndex_r4/Addressable Shift Register  infer_latency=on  depth=2  initVector=[0]  en=on  dbl_ovrd=off  use_behavioral_HDL=off  Optimization=Resource  use_rpm=off  block_type=addrsr
      settings: infoedit="Delay of  configurable length.  Any element  in the delay     line   can    be   addressed   and   driven    onto   the   output     port.<P><P>Hardware  notes: Implemented  using SRL16s.     If Virtex-4, Virtex-II or Spartan-3 devices are used, multiple SRLC16s are cascaded together."  xl_area=[225 0 0 450 0 0 0]  block_version=VER_STRING_GOES_HERE
  Delay1 : xbsIndex_r4/Delay  rst=off  infoeditControl=Selection of Reset will increase slice count due to use of real FFs and instead of SRLs  en=off  latency=1  dbl_ovrd=off  reg_retiming=off  block_type=delay
      settings: infoedit=Hardware notes: A delay line is a chain, each link of which is an SRL16 followed by a flip-flop. If register retiming is enabled, the delay line is a chain of flip-flops.  xl_area=[9 18 0 0 0 0 0]  block_version=VER_STRING_GOES_HERE
  ROM : xbsIndex_r4/ROM  depth=length(coef)  initVector=coef  distributed_mem=Block RAM  rst=off  init_reg=0  en=off  latency=1  gui_display_data_type=Fixed-point  arith_type="Signed  (2's comp)"  n_bits=coef_bit_width  bin_pt=coef_bin_pt  preci_type=Single  exp_width=8  frac_width=24  dbl_ovrd=off  optimize=Area  use_rpm=off  block_type=sprom
      settings: xl_area=[0 0 1 0 0 0 0]  block_version=VER_STRING_GOES_HERE
  Dout : Outport
  Coef Out : Outport  Port=2
  wires:
  en/1 -> Addressable Shift Register/3
  Din/1 -> Addressable Shift Register/1
  Addra/1 -> Addressable Shift Register/2
  Addressable Shift Register/1 -> Delay1/1
  Addrb/1 -> ROM/1
  ROM/1 -> Coef Out/1
  Delay1/1 -> Dout/1

== system sysgenDDC/DDC/H(z) Polyphase Decimator 2:1/2 Channel Decimate by 2 MAC FIR /Memory control ==
  Constant : xbsIndex_r4/Constant  const=length(coef)-4  gui_display_data_type=Fixed-point  arith_type=Unsigned  n_bits=ceil(log2(length(coef)-4))  bin_pt=0  preci_type=Single  exp_width=8  frac_width=24  explicit_period=off  period=1  equ=P=C  opselect=C  inp2=PCIN>>17  opr=+  inp1=P  carry=CIN  dbl_ovrd=off  block_type=constant
      settings: block_version=VER_STRING_GOES_HERE
  Counter1 : xbsIndex_r4/Counter  cnt_type=Count Limited  cnt_to=length(coef)-4  operation=Up  start_count=0  cnt_by_val=4  arith_type=Unsigned  n_bits=ceil(log2(length(coef)-1))  bin_pt=0  load_pin=off  rst=off  en=off  explicit_period=off  period=Ts/(length(coef)/2)  dbl_ovrd=off  use_behavioral_HDL=off  implementation=Fabric  use_rpm=off  block_type=counter
      settings: xl_area=[6 8 0 11 0 0 0]  block_version=VER_STRING_GOES_HERE
  Counter2 : xbsIndex_r4/Counter  cnt_type=Count Limited  cnt_to=length(coef)-1  operation=Up  start_count=0  cnt_by_val=1  arith_type=Unsigned  n_bits=ceil(log2(length(coef)-1))  bin_pt=0  load_pin=off  rst=off  en=off  explicit_period=off  period=Ts/(length(coef)/2)  dbl_ovrd=off  use_behavioral_HDL=off  implementation=Fabric  use_rpm=off  block_type=counter
      settings: xl_area=[6 8 0 11 0 0 0]  block_version=VER_STRING_GOES_HERE
  Relational : xbsIndex_r4/Relational  mode=a=b  en=off  latency=0  dbl_ovrd=off  block_type=relational
      settings: xl_area=[2 0 0 4 0 0 0]  block_version=VER_STRING_GOES_HERE
  Data Addr : Outport
  we : Outport  Port=2
  Coef Addr : Outport  Port=3
  wires:
  Counter1/1 -> Relational/1, Data Addr/1
  Constant/1 -> Relational/2
  Relational/1 -> we/1
  Counter2/1 -> Coef Addr/1
